simulink model "ddc_bpm_476_066"  (Simulink 7.8)
settings: Solver=ode45  StartTime=0.0  StopTime=2e-3  RelTol=1e-3
undefined symbols (not defined in the file): decim_factor_poly_35, dt_sim, frev_476, Fs_adc, n_ch, n_ovs, R_fofb, R_sec, R_sec_cfir, R_sec_pfir, xlipgetpartsetting
libraries: xbsIndex_r4 x1436, simulink x7
(part 2 of 12)

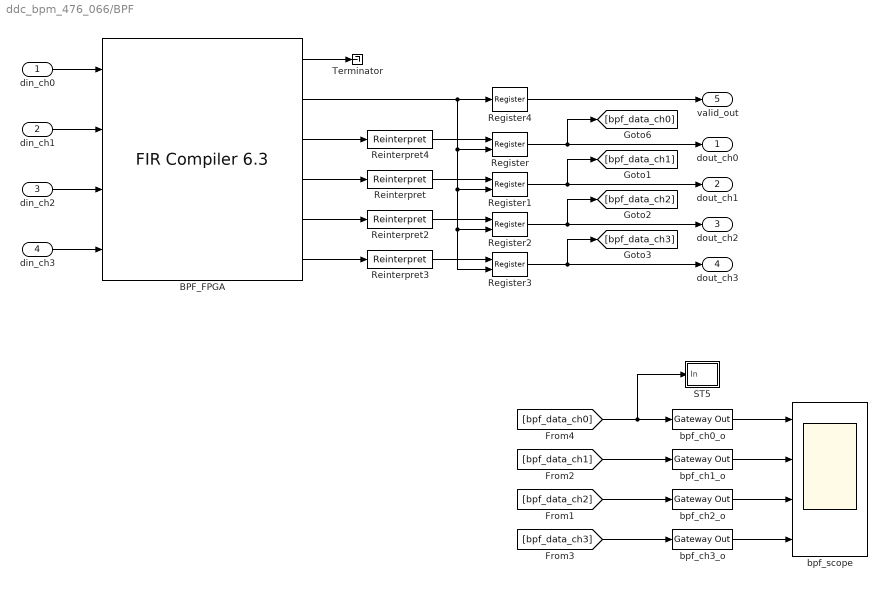
== system ddc_bpm_476_066/BPF ==
  din_ch0 : Inport
  din_ch1 : Inport  Port=2
  din_ch2 : Inport  Port=3
  din_ch3 : Inport  Port=4
  BPF_FPGA : xbsIndex_r4/FIR Compiler 6.3   coefficientvector=Hbpf_adc.Numerator  coefficient_sets=1  coefficient_reload=off  filter_type=Single_Rate  rate_change_type=Integer  interpolation_rate=1  decimation_rate=1  zero_pack_factor=1  channel_sequence=Basic  number_channels=1  pattern_list='P4-0,P4-1,P4-2,P4-3,P4-4'  number_paths=4  ratespecification=Hardware_Oversampling_Rate  sampleperiod=2  hardwareoversamplingrate=n_ovs  coefficient_sign=Signed  quantization=Quantize_Only  coefficient_width=16  bestprecision=on  coefficient_fractional_bits=17  coefficient_structure=Inferred  output_rounding_mode=Convergent_Rounding_to_Even  output_width=24  filter_architecture=Systolic_Multiply_Accumulate  optimization_goal=Area  data_buffer_type=Automatic  coefficient_buffer_type=Automatic  input_buffer_type=Automatic  output_buffer_type=Automatic  preference_for_other_storage=Automatic  multi_column_support=Automatic  columnconfig='10'  inter_column_pipe_length=4  data_has_tlast=Not_Required  m_data_has_tready=off  s_data_has_fifo=off  s_data_has_tuser=Not_Required  m_data_has_tuser=Not_Required  s_config_sync_mode=On_Vector  s_config_method=Single  num_reload_slots=1  has_aclken=off  has_aresetn=off  infoeditControl=ARESETn must be asserted for a minmum of 2 cycles  trim_axipin_name=on  passband_min=0.0  passband_max=0.5  stopband_min=0.5  stopband_max=1.0  filter_selection=1  gui_behaviour=Sysgen_GUI  data_sign=Signed  data_width=16  data_fractional_bits=0  data_tuser_width=1  wrapper_available=true  ip_wrap_arbitrary_binary_point=true  simulation_type=external_xfix  simulation_model=firv6_3_CModel:firv6_3_cmodel  ip_name=FIR Compiler  ip_version=6.3  dsptool_ready=true  ipcore_usecache=true  ipcore_useipmodelcache=true  ipcore_xco_need_fpga_part=true  port_translation_map={ 'aclken' => 'en', 'aresetn' => 'rst' }  run_core_at_system_period=true  ipcore_fpga_part=xlipgetpartsetting(gcb, {'virtex6', 'xc6vlx75t', '-3', 'ff784'})  block_type=fir_compiler_v6_3
      settings: infoedit=Maximum Possible : Maximizes oversampling rate. Abstracted input handshake (no s_data_tvalid) and automatic rate propagation.<br>Hardware Oversampling Rate : Specifies oversampling rate relative to the input sample period. Abstracted input handshake (no s_data_tvalid) and automatic rate propagation.<br>Sample Period : Specifies absolute oversampling rate. No input handshake abstraction (exposes s_data_tvalid) and no rate propagation.
  Register{,1..3} (4 alike) : xbsIndex_r4/Register  init=0  rst=off  en=on  dbl_ovrd=off  block_type=register
  Register4 : xbsIndex_r4/Register  init=0  rst=off  en=off  dbl_ovrd=off  block_type=register
  Reinterpret{,2..4} (4 alike) : xbsIndex_r4/Reinterpret  force_arith_type=off  arith_type=Unsigned  force_bin_pt=on  bin_pt=22  block_type=reinterpret
  ST5 : Subsystem
  Terminator : Terminator
  bpf_ch0_o : xbsIndex_r4/Gateway Out  inherit_from_input=on  hdl_port=on  timing_constraint=Data Rate  locs_specified=off  LOCs={}  UseAsDAC=off  DACChannel='1'  block_type=gatewayout
      settings: infoedit="Gateway out block.  Converts Xilinx fixed-point or floating-point type inputs into ouputs of type Simulink integer, single, double, or fixed point.<br><br>Hardware notes:  In hardware these blocks become top level output ports or are discarded, depending on how they are configured."
  bpf_ch1_o : xbsIndex_r4/Gateway Out  inherit_from_input=on  hdl_port=on  timing_constraint=Data Rate  locs_specified=off  LOCs={}  UseAsDAC=off  DACChannel='1'  block_type=gatewayout
      settings: infoedit="Gateway out block.  Converts Xilinx fixed-point or floating-point type inputs into ouputs of type Simulink integer, single, double, or fixed point.<br><br>Hardware notes:  In hardware these blocks become top level output ports or are discarded, depending on how they are configured."
  bpf_ch2_o : xbsIndex_r4/Gateway Out  inherit_from_input=on  hdl_port=on  timing_constraint=Data Rate  locs_specified=off  LOCs={}  UseAsDAC=off  DACChannel='1'  block_type=gatewayout
      settings: infoedit="Gateway out block.  Converts Xilinx fixed-point or floating-point type inputs into ouputs of type Simulink integer, single, double, or fixed point.<br><br>Hardware notes:  In hardware these blocks become top level output ports or are discarded, depending on how they are configured."
  bpf_ch3_o : xbsIndex_r4/Gateway Out  inherit_from_input=on  hdl_port=on  timing_constraint=Data Rate  locs_specified=off  LOCs={}  UseAsDAC=off  DACChannel='1'  block_type=gatewayout
      settings: infoedit="Gateway out block.  Converts Xilinx fixed-point or floating-point type inputs into ouputs of type Simulink integer, single, double, or fixed point.<br><br>Hardware notes:  In hardware these blocks become top level output ports or are discarded, depending on how they are configured."
  bpf_scope : Scope  NumInputPorts=4
      settings: TimeRange=0.00011214  YMin=-0.1~-1.5~-0.002~-1.5  YMax=1~1.5~0.00075~1.5  SaveName=ScopeData16  MaxDataPoints=1000000  SampleInput=on
  dout_ch0 : Outport
  dout_ch1 : Outport  Port=2
  dout_ch2 : Outport  Port=3
  dout_ch3 : Outport  Port=4
  valid_out : Outport  Port=5
  wires:
  din_ch0/1 -> BPF_FPGA/1
  BPF_FPGA/1 -> Terminator/1
  BPF_FPGA/2 -> Register/2, Register1/2, Register2/2, Register3/2, Register4/1
  BPF_FPGA/3 -> Reinterpret4/1
  BPF_FPGA/5 -> Reinterpret2/1
  din_ch1/1 -> BPF_FPGA/2
  BPF_FPGA/4 -> Reinterpret/1
  bpf_ch3_o/1 -> bpf_scope/4
  bpf_ch2_o/1 -> bpf_scope/3
  bpf_ch1_o/1 -> bpf_scope/2
  bpf_ch0_o/1 -> bpf_scope/1
  din_ch2/1 -> BPF_FPGA/3
  din_ch3/1 -> BPF_FPGA/4
  BPF_FPGA/6 -> Reinterpret3/1
  [bpf_data_ch0] -> bpf_ch0_o/1, ST5/1(In)
  [bpf_data_ch1] -> bpf_ch1_o/1
  [bpf_data_ch3] -> bpf_ch3_o/1
  [bpf_data_ch2] -> bpf_ch2_o/1
  Register/1 -> dout_ch0/1, [bpf_data_ch0]
  Register1/1 -> dout_ch1/1, [bpf_data_ch1]
  Reinterpret4/1 -> Register/1
  Reinterpret/1 -> Register1/1
  Reinterpret2/1 -> Register2/1
  Reinterpret3/1 -> Register3/1
  Register2/1 -> dout_ch2/1, [bpf_data_ch2]
  Register3/1 -> dout_ch3/1, [bpf_data_ch3]
  Register4/1 -> valid_out/1

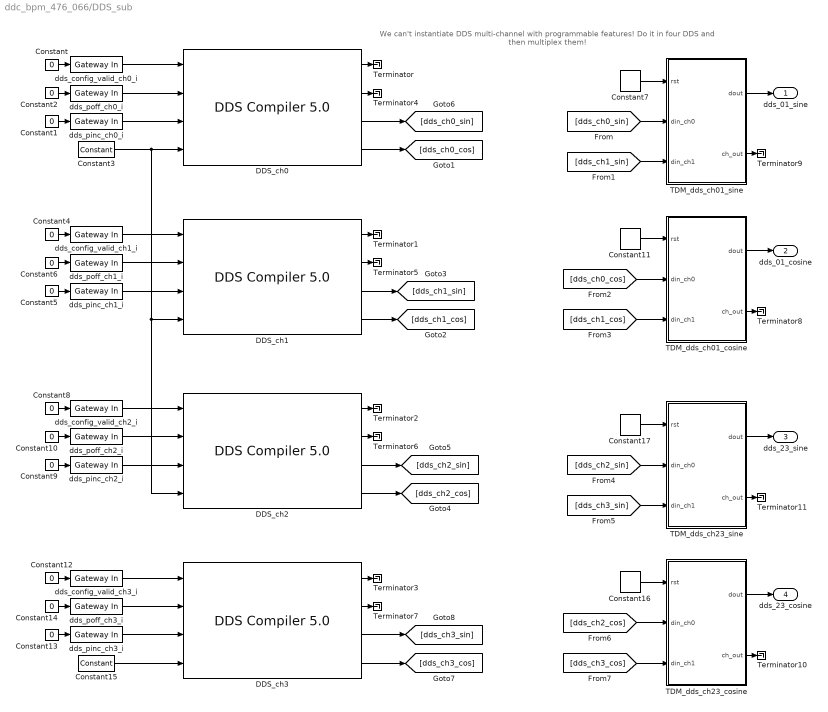
== system ddc_bpm_476_066/DDS_sub ==
  note: We can't instantiate DDS multi-channel with programmable features!
      | Do it in four DDS and then multiplex them!
  Constant{,1..2,4..6,8..10,12..14} (12 alike) : Constant  Value=0
  Constant{7,11,16..17} (4 alike) : xbsIndex_r4/Constant  const=0  gui_display_data_type=Boolean  arith_type=Boolean  n_bits=16  bin_pt=14  preci_type=Single  exp_width=8  frac_width=24  explicit_period=on  period=1/Fs_adc/n_ovs  equ=P=C  opselect=C  inp2=PCIN>>17  opr=+  inp1=P  carry=CIN  dbl_ovrd=off  block_type=constant
  Constant15 : xbsIndex_r4/Constant  const=1  gui_display_data_type=Boolean  arith_type=Boolean  n_bits=24  bin_pt=22  preci_type=Single  exp_width=8  frac_width=24  explicit_period=on  period=1/Fs_adc  equ=P=C  opselect=C  inp2=PCIN>>17  opr=+  inp1=P  carry=CIN  dbl_ovrd=off  block_type=constant
  Constant3 : xbsIndex_r4/Constant  const=1  gui_display_data_type=Boolean  arith_type=Boolean  n_bits=24  bin_pt=22  preci_type=Single  exp_width=8  frac_width=24  explicit_period=on  period=1/Fs_adc  equ=P=C  opselect=C  inp2=PCIN>>17  opr=+  inp1=P  carry=CIN  dbl_ovrd=off  block_type=constant
  DDS_ch{0..3} (4 alike) : xbsIndex_r4/DDS Compiler 5.0   partspresent=Phase_Generator_and_SIN_COS_LUT  dds_clock_rate=Fs_adc/1e6  channels=1  parameter_entry=Hardware_Parameters  spurious_free_dynamic_range=36  frequency_resolution=0.4  noise_shaping=Taylor_Series_Corrected  phase_width=30  output_width=24  output_selection=Sine_and_Cosine  negative_sine=on  negative_cosine=off  amplitude_mode=Unit_Circle  memory_type=Auto  optimization_goal=Auto  dsp48_use=Minimal  latency_configuration=Auto  latency=12  has_phase_out=off  has_aclken=off  has_aresetn=off  explicit_period=on  period=1/Fs_adc  data_has_tlast=Not_Required  has_tready=on  s_phase_has_tuser=Not_Required  m_data_has_tuser=Not_Required  m_phase_has_tuser=Not_Required  s_phase_tuser_width=1  s_config_sync_mode=On_Vector  phase_increment=Programmable  output_frequency1=0  output_frequency2=0  output_frequency3=0  output_frequency4=0  output_frequency5=0  output_frequency6=0  output_frequency7=0  output_frequency8=0  output_frequency9=0  output_frequency10=0  output_frequency11=0  output_frequency12=0  output_frequency13=0  output_frequency14=0  output_frequency15=0  output_frequency16=0  pinc1=dds_freq_bin  pinc2='0'  pinc3='0'  pinc4='0'  pinc5='0'  pinc6='0'  pinc7='0'  pinc8='0'  pinc9='0'  pinc10='0'  pinc11='0'  pinc12='0'  pinc13='0'  pinc14='0'  pinc15='0'  pinc16='0'  phase_offset=Programmable  phase_offset_angles1=0  phase_offset_angles2=0  phase_offset_angles3=0  phase_offset_angles4=0  phase_offset_angles5=0  phase_offset_angles6=0  phase_offset_angles7=0  phase_offset_angles8=0  phase_offset_angles9=0  phase_offset_angles10=0  phase_offset_angles11=0  phase_offset_angles12=0  phase_offset_angles13=0  phase_offset_angles14=0  phase_offset_angles15=0  phase_offset_angles16=0  poff1='0'  poff2='0'  poff3='0'  poff4='0'  poff5='0'  poff6='0'  poff7='0'  poff8='0'  poff9='0'  poff10='0'  poff11='0'  poff12='0'  poff13='0'  poff14='0'  poff15='0'  poff16='0'  trim_axipin_name=on  por_mode=false  gui_behaviour=Sysgen  ip_name=DDS Compiler  ip_version=5.0  dsptool_ready=true  wrapper_available=true  port_translation_map={ 'aclken' => 'en', 'aresetn' => 'rst' }  ipcore_xco_need_fpga_part=true  ipcore_fpga_part=xlipgetpartsetting(gcb, {'virtex6', 'xc6vlx75t', '-3', 'ff784'})  ipcore_usecache=true  ipcore_useipmodelcache=true  ipcore_verbose=false  block_type=dds_compiler_v5_0
  TDM_dds_ch01_cosine : Subsystem
  TDM_dds_ch01_sine : Subsystem
  TDM_dds_ch23_cosine : Subsystem
  TDM_dds_ch23_sine : Subsystem
  Terminator{,1..11} (12 alike) : Terminator
  dds_config_valid_ch0_i : xbsIndex_r4/Gateway In  gui_display_data_type=Boolean  arith_type=Boolean  n_bits=16  bin_pt=15  preci_type=Single  exp_width=8  frac_width=24  quantization=Truncate  overflow=Flag as error  period=1/Fs_adc  dbl_ovrd=off  timing_constraint=None  locs_specified=off  LOCs={}  inherit_from_input=off  UseAsADC=off  ADCChannel='1'  hdl_port=on  block_type=gatewayin
      settings: infoedit="Gateway in block.  Converts inputs of type Simulink integer, single, double and fixed point to  Xilinx fixed-point or floating-point data type.<br><br>Hardware notes:  In hardware these blocks become top level input ports."
  dds_config_valid_ch1_i : xbsIndex_r4/Gateway In  gui_display_data_type=Boolean  arith_type=Boolean  n_bits=16  bin_pt=15  preci_type=Single  exp_width=8  frac_width=24  quantization=Truncate  overflow=Flag as error  period=1/Fs_adc  dbl_ovrd=off  timing_constraint=None  locs_specified=off  LOCs={}  inherit_from_input=off  UseAsADC=off  ADCChannel='1'  hdl_port=on  block_type=gatewayin
      settings: infoedit="Gateway in block.  Converts inputs of type Simulink integer, single, double and fixed point to  Xilinx fixed-point or floating-point data type.<br><br>Hardware notes:  In hardware these blocks become top level input ports."
  dds_config_valid_ch2_i : xbsIndex_r4/Gateway In  gui_display_data_type=Boolean  arith_type=Boolean  n_bits=16  bin_pt=15  preci_type=Single  exp_width=8  frac_width=24  quantization=Truncate  overflow=Flag as error  period=1/Fs_adc  dbl_ovrd=off  timing_constraint=None  locs_specified=off  LOCs={}  inherit_from_input=off  UseAsADC=off  ADCChannel='1'  hdl_port=on  block_type=gatewayin
      settings: infoedit="Gateway in block.  Converts inputs of type Simulink integer, single, double and fixed point to  Xilinx fixed-point or floating-point data type.<br><br>Hardware notes:  In hardware these blocks become top level input ports."
  dds_config_valid_ch3_i : xbsIndex_r4/Gateway In  gui_display_data_type=Boolean  arith_type=Boolean  n_bits=16  bin_pt=15  preci_type=Single  exp_width=8  frac_width=24  quantization=Truncate  overflow=Flag as error  period=1/Fs_adc  dbl_ovrd=off  timing_constraint=None  locs_specified=off  LOCs={}  inherit_from_input=off  UseAsADC=off  ADCChannel='1'  hdl_port=on  block_type=gatewayin
      settings: infoedit="Gateway in block.  Converts inputs of type Simulink integer, single, double and fixed point to  Xilinx fixed-point or floating-point data type.<br><br>Hardware notes:  In hardware these blocks become top level input ports."
  dds_pinc_ch0_i : xbsIndex_r4/Gateway In  gui_display_data_type=Fixed-point  arith_type="Signed  (2's comp)"  n_bits=30  bin_pt=30  preci_type=Single  exp_width=8  frac_width=24  quantization=Truncate  overflow=Flag as error  period=1/Fs_adc  dbl_ovrd=off  timing_constraint=None  locs_specified=off  LOCs={}  inherit_from_input=off  UseAsADC=off  ADCChannel='1'  hdl_port=on  block_type=gatewayin
      settings: infoedit="Gateway in block.  Converts inputs of type Simulink integer, single, double and fixed point to  Xilinx fixed-point or floating-point data type.<br><br>Hardware notes:  In hardware these blocks become top level input ports."
  dds_pinc_ch1_i : xbsIndex_r4/Gateway In  gui_display_data_type=Fixed-point  arith_type="Signed  (2's comp)"  n_bits=30  bin_pt=30  preci_type=Single  exp_width=8  frac_width=24  quantization=Truncate  overflow=Flag as error  period=1/Fs_adc  dbl_ovrd=off  timing_constraint=None  locs_specified=off  LOCs={}  inherit_from_input=off  UseAsADC=off  ADCChannel='1'  hdl_port=on  block_type=gatewayin
      settings: infoedit="Gateway in block.  Converts inputs of type Simulink integer, single, double and fixed point to  Xilinx fixed-point or floating-point data type.<br><br>Hardware notes:  In hardware these blocks become top level input ports."
  dds_pinc_ch2_i : xbsIndex_r4/Gateway In  gui_display_data_type=Fixed-point  arith_type="Signed  (2's comp)"  n_bits=30  bin_pt=30  preci_type=Single  exp_width=8  frac_width=24  quantization=Truncate  overflow=Flag as error  period=1/Fs_adc  dbl_ovrd=off  timing_constraint=None  locs_specified=off  LOCs={}  inherit_from_input=off  UseAsADC=off  ADCChannel='1'  hdl_port=on  block_type=gatewayin
      settings: infoedit="Gateway in block.  Converts inputs of type Simulink integer, single, double and fixed point to  Xilinx fixed-point or floating-point data type.<br><br>Hardware notes:  In hardware these blocks become top level input ports."
  dds_pinc_ch3_i : xbsIndex_r4/Gateway In  gui_display_data_type=Fixed-point  arith_type="Signed  (2's comp)"  n_bits=30  bin_pt=30  preci_type=Single  exp_width=8  frac_width=24  quantization=Truncate  overflow=Flag as error  period=1/Fs_adc  dbl_ovrd=off  timing_constraint=None  locs_specified=off  LOCs={}  inherit_from_input=off  UseAsADC=off  ADCChannel='1'  hdl_port=on  block_type=gatewayin
      settings: infoedit="Gateway in block.  Converts inputs of type Simulink integer, single, double and fixed point to  Xilinx fixed-point or floating-point data type.<br><br>Hardware notes:  In hardware these blocks become top level input ports."
  dds_poff_ch0_i : xbsIndex_r4/Gateway In  gui_display_data_type=Fixed-point  arith_type="Signed  (2's comp)"  n_bits=30  bin_pt=30  preci_type=Single  exp_width=8  frac_width=24  quantization=Truncate  overflow=Flag as error  period=1/Fs_adc  dbl_ovrd=off  timing_constraint=None  locs_specified=off  LOCs={}  inherit_from_input=off  UseAsADC=off  ADCChannel='1'  hdl_port=on  block_type=gatewayin
      settings: infoedit="Gateway in block.  Converts inputs of type Simulink integer, single, double and fixed point to  Xilinx fixed-point or floating-point data type.<br><br>Hardware notes:  In hardware these blocks become top level input ports."
  dds_poff_ch1_i : xbsIndex_r4/Gateway In  gui_display_data_type=Fixed-point  arith_type="Signed  (2's comp)"  n_bits=30  bin_pt=30  preci_type=Single  exp_width=8  frac_width=24  quantization=Truncate  overflow=Flag as error  period=1/Fs_adc  dbl_ovrd=off  timing_constraint=None  locs_specified=off  LOCs={}  inherit_from_input=off  UseAsADC=off  ADCChannel='1'  hdl_port=on  block_type=gatewayin
      settings: infoedit="Gateway in block.  Converts inputs of type Simulink integer, single, double and fixed point to  Xilinx fixed-point or floating-point data type.<br><br>Hardware notes:  In hardware these blocks become top level input ports."
  dds_poff_ch2_i : xbsIndex_r4/Gateway In  gui_display_data_type=Fixed-point  arith_type="Signed  (2's comp)"  n_bits=30  bin_pt=30  preci_type=Single  exp_width=8  frac_width=24  quantization=Truncate  overflow=Flag as error  period=1/Fs_adc  dbl_ovrd=off  timing_constraint=None  locs_specified=off  LOCs={}  inherit_from_input=off  UseAsADC=off  ADCChannel='1'  hdl_port=on  block_type=gatewayin
      settings: infoedit="Gateway in block.  Converts inputs of type Simulink integer, single, double and fixed point to  Xilinx fixed-point or floating-point data type.<br><br>Hardware notes:  In hardware these blocks become top level input ports."
  dds_poff_ch3_i : xbsIndex_r4/Gateway In  gui_display_data_type=Fixed-point  arith_type="Signed  (2's comp)"  n_bits=30  bin_pt=30  preci_type=Single  exp_width=8  frac_width=24  quantization=Truncate  overflow=Flag as error  period=1/Fs_adc  dbl_ovrd=off  timing_constraint=None  locs_specified=off  LOCs={}  inherit_from_input=off  UseAsADC=off  ADCChannel='1'  hdl_port=on  block_type=gatewayin
      settings: infoedit="Gateway in block.  Converts inputs of type Simulink integer, single, double and fixed point to  Xilinx fixed-point or floating-point data type.<br><br>Hardware notes:  In hardware these blocks become top level input ports."
  dds_01_sine : Outport
  dds_01_cosine : Outport  Port=2
  dds_23_sine : Outport  Port=3
  dds_23_cosine : Outport  Port=4
  wires:
  Constant3/1 -> DDS_ch0/4, DDS_ch1/4, DDS_ch2/4
  dds_poff_ch0_i/1 -> DDS_ch0/2
  dds_pinc_ch0_i/1 -> DDS_ch0/3
  dds_config_valid_ch0_i/1 -> DDS_ch0/1
  DDS_ch0/1 -> Terminator/1
  Constant/1 -> dds_config_valid_ch0_i/1
  Constant1/1 -> dds_pinc_ch0_i/1
  Constant2/1 -> dds_poff_ch0_i/1
  dds_poff_ch1_i/1 -> DDS_ch1/2
  dds_pinc_ch1_i/1 -> DDS_ch1/3
  dds_config_valid_ch1_i/1 -> DDS_ch1/1
  DDS_ch1/1 -> Terminator1/1
  Constant4/1 -> dds_config_valid_ch1_i/1
  Constant5/1 -> dds_pinc_ch1_i/1
  Constant6/1 -> dds_poff_ch1_i/1
  dds_poff_ch2_i/1 -> DDS_ch2/2
  dds_pinc_ch2_i/1 -> DDS_ch2/3
  dds_config_valid_ch2_i/1 -> DDS_ch2/1
  DDS_ch2/1 -> Terminator2/1
  Constant8/1 -> dds_config_valid_ch2_i/1
  Constant9/1 -> dds_pinc_ch2_i/1
  Constant10/1 -> dds_poff_ch2_i/1
  Constant15/1 -> DDS_ch3/4
  dds_poff_ch3_i/1 -> DDS_ch3/2
  dds_pinc_ch3_i/1 -> DDS_ch3/3
  dds_config_valid_ch3_i/1 -> DDS_ch3/1
  DDS_ch3/1 -> Terminator3/1
  Constant12/1 -> dds_config_valid_ch3_i/1
  Constant13/1 -> dds_pinc_ch3_i/1
  Constant14/1 -> dds_poff_ch3_i/1
  Constant7/1 -> TDM_dds_ch01_sine/1(rst)
  TDM_dds_ch01_sine/1(dout) -> dds_01_sine/1
  Constant11/1 -> TDM_dds_ch01_cosine/1(rst)
  TDM_dds_ch01_cosine/1(dout) -> dds_01_cosine/1
  DDS_ch0/3 -> [dds_ch0_sin]
  DDS_ch0/4 -> [dds_ch0_cos]
  DDS_ch1/3 -> [dds_ch1_sin]
  DDS_ch1/4 -> [dds_ch1_cos]
  DDS_ch2/3 -> [dds_ch2_sin]
  DDS_ch2/4 -> [dds_ch2_cos]
  DDS_ch3/3 -> [dds_ch3_sin]
  DDS_ch3/4 -> [dds_ch3_cos]
  [dds_ch0_sin] -> TDM_dds_ch01_sine/2(din_ch0)
  [dds_ch1_sin] -> TDM_dds_ch01_sine/3(din_ch1)
  [dds_ch0_cos] -> TDM_dds_ch01_cosine/2(din_ch0)
  [dds_ch1_cos] -> TDM_dds_ch01_cosine/3(din_ch1)
  Constant17/1 -> TDM_dds_ch23_sine/1(rst)
  TDM_dds_ch23_sine/1(dout) -> dds_23_sine/1
  Constant16/1 -> TDM_dds_ch23_cosine/1(rst)
  TDM_dds_ch23_cosine/1(dout) -> dds_23_cosine/1
  [dds_ch2_sin] -> TDM_dds_ch23_sine/2(din_ch0)
  [dds_ch3_sin] -> TDM_dds_ch23_sine/3(din_ch1)
  [dds_ch2_cos] -> TDM_dds_ch23_cosine/2(din_ch0)
  [dds_ch3_cos] -> TDM_dds_ch23_cosine/3(din_ch1)
  DDS_ch0/2 -> Terminator4/1
  DDS_ch1/2 -> Terminator5/1
  DDS_ch2/2 -> Terminator6/1
  DDS_ch3/2 -> Terminator7/1
  TDM_dds_ch01_cosine/2(ch_out) -> Terminator8/1
  TDM_dds_ch01_sine/2(ch_out) -> Terminator9/1
  TDM_dds_ch23_cosine/2(ch_out) -> Terminator10/1
  TDM_dds_ch23_sine/2(ch_out) -> Terminator11/1

== system ddc_bpm_476_066/FOFB_amp ==
  Q_in0 : Inport
  I_in0 : Inport  Port=2
  ch_in0 : Inport  Port=3
  Q_in1 : Inport  Port=4
  I_in1 : Inport  Port=5
  ch_in1 : Inport  Port=6
  ST1 : Subsystem
  ST5 : Subsystem
  TDDM_fofb_amp_4ch : Subsystem
  Terminator{,1..3} (4 alike) : Terminator
  fofb_amp0 : Subsystem
  fofb_amp1 : Subsystem
  amp_out0 : Outport
  amp_out1 : Outport  Port=2
  amp_out2 : Outport  Port=3
  amp_out3 : Outport  Port=4
  wires:
  Q_in0/1 -> fofb_amp0/1(Q_in)
  I_in0/1 -> fofb_amp0/2(I_in)
  ch_in0/1 -> fofb_amp0/3(ch_in)
  Q_in1/1 -> fofb_amp1/1(Q_in)
  I_in1/1 -> fofb_amp1/2(I_in)
  ch_in1/1 -> fofb_amp1/3(ch_in)
  TDDM_fofb_amp_4ch/1(amp_out0) -> amp_out0/1, ST1/1(In)
  TDDM_fofb_amp_4ch/2(amp_out1) -> amp_out1/1
  TDDM_fofb_amp_4ch/3(amp_out2) -> amp_out2/1
  TDDM_fofb_amp_4ch/4(amp_out3) -> amp_out3/1
  fofb_amp0/1(amp_out) -> TDDM_fofb_amp_4ch/1(amp_in0), ST5/1(In)
  fofb_amp0/4(ch_out) -> TDDM_fofb_amp_4ch/2(ch_in0)
  fofb_amp1/1(amp_out) -> TDDM_fofb_amp_4ch/3(amp_in1)
  fofb_amp1/4(ch_out) -> TDDM_fofb_amp_4ch/4(ch_in1)
  fofb_amp0/2(phase_out) -> Terminator/1
  fofb_amp0/3(valid_out) -> Terminator1/1
  fofb_amp1/2(phase_out) -> Terminator2/1
  fofb_amp1/3(valid_out) -> Terminator3/1

== system ddc_bpm_476_066/K_fofb_mult3 ==
  In1 : Inport
  In2 : Inport  Port=2
  vld_in : Inport  Port=3
  Cast_truncate1 : Subsystem
  Delay1 : xbsIndex_r4/Delay  rst=off  infoeditControl=Selection of Reset will increase slice count due to use of real FFs and instead of SRLs  en=off  latency=9  dbl_ovrd=off  reg_retiming=off  block_type=delay
  Kx_tbt : xbsIndex_r4/Mult  precision=Full  arith_type="Signed  (2's comp)"  n_bits=16  bin_pt=14  quantization=Truncate  overflow=Wrap  en=off  latency=8  dbl_ovrd=off  use_behavioral_HDL=off  opt=Speed  use_embedded=off  optimum_pipeline=on  pipeline=on  use_rpm=on  placement_style=Triangular  block_type=mult
  Register : xbsIndex_r4/Register  init=0  rst=off  en=off  dbl_ovrd=off  block_type=register
  Out1 : Outport
  vld_out : Outport  Port=2
  wires:
  Kx_tbt/1 -> Cast_truncate1/1(In1)
  In1/1 -> Kx_tbt/1
  Cast_truncate1/1(Out1) -> Register/1
  In2/1 -> Kx_tbt/2
  Register/1 -> Out1/1
  vld_in/1 -> Delay1/1
  Delay1/1 -> vld_out/1

== system ddc_bpm_476_066/K_fofb_mult4 ==
  In1 : Inport
  In2 : Inport  Port=2
  vld_in : Inport  Port=3
  Cast_truncate1 : Subsystem
  Delay1 : xbsIndex_r4/Delay  rst=off  infoeditControl=Selection of Reset will increase slice count due to use of real FFs and instead of SRLs  en=off  latency=9  dbl_ovrd=off  reg_retiming=off  block_type=delay
  Kx_tbt : xbsIndex_r4/Mult  precision=Full  arith_type="Signed  (2's comp)"  n_bits=16  bin_pt=14  quantization=Truncate  overflow=Wrap  en=off  latency=8  dbl_ovrd=off  use_behavioral_HDL=off  opt=Speed  use_embedded=off  optimum_pipeline=on  pipeline=on  use_rpm=on  placement_style=Triangular  block_type=mult
  Register : xbsIndex_r4/Register  init=0  rst=off  en=off  dbl_ovrd=off  block_type=register
  Out1 : Outport
  vld_out : Outport  Port=2
  wires:
  Kx_tbt/1 -> Cast_truncate1/1(In1)
  In1/1 -> Kx_tbt/1
  Cast_truncate1/1(Out1) -> Register/1
  In2/1 -> Kx_tbt/2
  Register/1 -> Out1/1
  vld_in/1 -> Delay1/1
  Delay1/1 -> vld_out/1

== system ddc_bpm_476_066/K_fofb_mult5 ==
  In1 : Inport
  In2 : Inport  Port=2
  vld_in : Inport  Port=3
  Cast_truncate1 : Subsystem
  Delay1 : xbsIndex_r4/Delay  rst=off  infoeditControl=Selection of Reset will increase slice count due to use of real FFs and instead of SRLs  en=off  latency=9  dbl_ovrd=off  reg_retiming=off  block_type=delay
  Kx_tbt : xbsIndex_r4/Mult  precision=Full  arith_type="Signed  (2's comp)"  n_bits=16  bin_pt=14  quantization=Truncate  overflow=Wrap  en=off  latency=8  dbl_ovrd=off  use_behavioral_HDL=off  opt=Speed  use_embedded=off  optimum_pipeline=on  pipeline=on  use_rpm=on  placement_style=Triangular  block_type=mult
  Register : xbsIndex_r4/Register  init=0  rst=off  en=off  dbl_ovrd=off  block_type=register
  Out1 : Outport
  vld_out : Outport  Port=2
  wires:
  Kx_tbt/1 -> Cast_truncate1/1(In1)
  In1/1 -> Kx_tbt/1
  Cast_truncate1/1(Out1) -> Register/1
  In2/1 -> Kx_tbt/2
  Register/1 -> Out1/1
  vld_in/1 -> Delay1/1
  Delay1/1 -> vld_out/1

== system ddc_bpm_476_066/K_monit_1_mult ==
  In1 : Inport
  In2 : Inport  Port=2
  vld_in : Inport  Port=3
  Cast_truncate1 : Subsystem
  Delay1 : xbsIndex_r4/Delay  rst=off  infoeditControl=Selection of Reset will increase slice count due to use of real FFs and instead of SRLs  en=off  latency=9  dbl_ovrd=off  reg_retiming=off  block_type=delay
  Kx_tbt : xbsIndex_r4/Mult  precision=Full  arith_type="Signed  (2's comp)"  n_bits=16  bin_pt=14  quantization=Truncate  overflow=Wrap  en=off  latency=8  dbl_ovrd=off  use_behavioral_HDL=off  opt=Speed  use_embedded=off  optimum_pipeline=on  pipeline=on  use_rpm=on  placement_style=Triangular  block_type=mult
  Register : xbsIndex_r4/Register  init=0  rst=off  en=off  dbl_ovrd=off  block_type=register
  Out1 : Outport
  vld_out : Outport  Port=2
  wires:
  Kx_tbt/1 -> Cast_truncate1/1(In1)
  In1/1 -> Kx_tbt/1
  Cast_truncate1/1(Out1) -> Register/1
  In2/1 -> Kx_tbt/2
  Register/1 -> Out1/1
  vld_in/1 -> Delay1/1
  Delay1/1 -> vld_out/1

== system ddc_bpm_476_066/K_monit_1_mult2 ==
  In1 : Inport
  In2 : Inport  Port=2
  vld_in : Inport  Port=3
  Cast_truncate1 : Subsystem
  Delay1 : xbsIndex_r4/Delay  rst=off  infoeditControl=Selection of Reset will increase slice count due to use of real FFs and instead of SRLs  en=off  latency=9  dbl_ovrd=off  reg_retiming=off  block_type=delay
  Kx_tbt : xbsIndex_r4/Mult  precision=Full  arith_type="Signed  (2's comp)"  n_bits=16  bin_pt=14  quantization=Truncate  overflow=Wrap  en=off  latency=8  dbl_ovrd=off  use_behavioral_HDL=off  opt=Speed  use_embedded=off  optimum_pipeline=on  pipeline=on  use_rpm=on  placement_style=Triangular  block_type=mult
  Register : xbsIndex_r4/Register  init=0  rst=off  en=off  dbl_ovrd=off  block_type=register
  Out1 : Outport
  vld_out : Outport  Port=2
  wires:
  Kx_tbt/1 -> Cast_truncate1/1(In1)
  In1/1 -> Kx_tbt/1
  Cast_truncate1/1(Out1) -> Register/1
  In2/1 -> Kx_tbt/2
  Register/1 -> Out1/1
  vld_in/1 -> Delay1/1
  Delay1/1 -> vld_out/1

== system ddc_bpm_476_066/K_monit_1_mult6 ==
  In1 : Inport
  In2 : Inport  Port=2
  vld_in : Inport  Port=3
  Cast_truncate1 : Subsystem
  Delay1 : xbsIndex_r4/Delay  rst=off  infoeditControl=Selection of Reset will increase slice count due to use of real FFs and instead of SRLs  en=off  latency=9  dbl_ovrd=off  reg_retiming=off  block_type=delay
  Kx_tbt : xbsIndex_r4/Mult  precision=Full  arith_type="Signed  (2's comp)"  n_bits=16  bin_pt=14  quantization=Truncate  overflow=Wrap  en=off  latency=8  dbl_ovrd=off  use_behavioral_HDL=off  opt=Speed  use_embedded=off  optimum_pipeline=on  pipeline=on  use_rpm=on  placement_style=Triangular  block_type=mult
  Register : xbsIndex_r4/Register  init=0  rst=off  en=off  dbl_ovrd=off  block_type=register
  Out1 : Outport
  vld_out : Outport  Port=2
  wires:
  Kx_tbt/1 -> Cast_truncate1/1(In1)
  In1/1 -> Kx_tbt/1
  Cast_truncate1/1(Out1) -> Register/1
  In2/1 -> Kx_tbt/2
  Register/1 -> Out1/1
  vld_in/1 -> Delay1/1
  Delay1/1 -> vld_out/1

== system ddc_bpm_476_066/K_monit_mult3 ==
  In1 : Inport
  In2 : Inport  Port=2
  vld_in : Inport  Port=3
  Cast_truncate1 : Subsystem
  Delay1 : xbsIndex_r4/Delay  rst=off  infoeditControl=Selection of Reset will increase slice count due to use of real FFs and instead of SRLs  en=off  latency=9  dbl_ovrd=off  reg_retiming=off  block_type=delay
  Kx_tbt : xbsIndex_r4/Mult  precision=Full  arith_type="Signed  (2's comp)"  n_bits=16  bin_pt=14  quantization=Truncate  overflow=Wrap  en=off  latency=8  dbl_ovrd=off  use_behavioral_HDL=off  opt=Speed  use_embedded=off  optimum_pipeline=on  pipeline=on  use_rpm=on  placement_style=Triangular  block_type=mult
  Register : xbsIndex_r4/Register  init=0  rst=off  en=off  dbl_ovrd=off  block_type=register
  Out1 : Outport
  vld_out : Outport  Port=2
  wires:
  Kx_tbt/1 -> Cast_truncate1/1(In1)
  In1/1 -> Kx_tbt/1
  Cast_truncate1/1(Out1) -> Register/1
  In2/1 -> Kx_tbt/2
  Register/1 -> Out1/1
  vld_in/1 -> Delay1/1
  Delay1/1 -> vld_out/1

== system ddc_bpm_476_066/K_monit_mult4 ==
  In1 : Inport
  In2 : Inport  Port=2
  vld_in : Inport  Port=3
  Cast_truncate1 : Subsystem
  Delay1 : xbsIndex_r4/Delay  rst=off  infoeditControl=Selection of Reset will increase slice count due to use of real FFs and instead of SRLs  en=off  latency=9  dbl_ovrd=off  reg_retiming=off  block_type=delay
  Kx_tbt : xbsIndex_r4/Mult  precision=Full  arith_type="Signed  (2's comp)"  n_bits=16  bin_pt=14  quantization=Truncate  overflow=Wrap  en=off  latency=8  dbl_ovrd=off  use_behavioral_HDL=off  opt=Speed  use_embedded=off  optimum_pipeline=on  pipeline=on  use_rpm=on  placement_style=Triangular  block_type=mult
  Register : xbsIndex_r4/Register  init=0  rst=off  en=off  dbl_ovrd=off  block_type=register
  Out1 : Outport
  vld_out : Outport  Port=2
  wires:
  Kx_tbt/1 -> Cast_truncate1/1(In1)
  In1/1 -> Kx_tbt/1
  Cast_truncate1/1(Out1) -> Register/1
  In2/1 -> Kx_tbt/2
  Register/1 -> Out1/1
  vld_in/1 -> Delay1/1
  Delay1/1 -> vld_out/1

== system ddc_bpm_476_066/K_monit_mult5 ==
  In1 : Inport
  In2 : Inport  Port=2
  vld_in : Inport  Port=3
  Cast_truncate1 : Subsystem
  Delay1 : xbsIndex_r4/Delay  rst=off  infoeditControl=Selection of Reset will increase slice count due to use of real FFs and instead of SRLs  en=off  latency=9  dbl_ovrd=off  reg_retiming=off  block_type=delay
  Kx_tbt : xbsIndex_r4/Mult  precision=Full  arith_type="Signed  (2's comp)"  n_bits=16  bin_pt=14  quantization=Truncate  overflow=Wrap  en=off  latency=8  dbl_ovrd=off  use_behavioral_HDL=off  opt=Speed  use_embedded=off  optimum_pipeline=on  pipeline=on  use_rpm=on  placement_style=Triangular  block_type=mult
  Register : xbsIndex_r4/Register  init=0  rst=off  en=off  dbl_ovrd=off  block_type=register
  Out1 : Outport
  vld_out : Outport  Port=2
  wires:
  Kx_tbt/1 -> Cast_truncate1/1(In1)
  In1/1 -> Kx_tbt/1
  Cast_truncate1/1(Out1) -> Register/1
  In2/1 -> Kx_tbt/2
  Register/1 -> Out1/1
  vld_in/1 -> Delay1/1
  Delay1/1 -> vld_out/1

== system ddc_bpm_476_066/K_tbt_mult ==
  In1 : Inport
  In2 : Inport  Port=2
  vld_in : Inport  Port=3
  Cast_truncate1 : Subsystem
  Delay1 : xbsIndex_r4/Delay  rst=off  infoeditControl=Selection of Reset will increase slice count due to use of real FFs and instead of SRLs  en=off  latency=9  dbl_ovrd=off  reg_retiming=off  block_type=delay
  Kx_tbt : xbsIndex_r4/Mult  precision=Full  arith_type="Signed  (2's comp)"  n_bits=16  bin_pt=14  quantization=Truncate  overflow=Wrap  en=off  latency=8  dbl_ovrd=off  use_behavioral_HDL=off  opt=Speed  use_embedded=off  optimum_pipeline=on  pipeline=on  use_rpm=on  placement_style=Triangular  block_type=mult
  Register : xbsIndex_r4/Register  init=0  rst=off  en=off  dbl_ovrd=off  block_type=register
  Out1 : Outport
  vld_out : Outport  Port=2
  wires:
  Kx_tbt/1 -> Cast_truncate1/1(In1)
  In1/1 -> Kx_tbt/1
  Cast_truncate1/1(Out1) -> Register/1
  In2/1 -> Kx_tbt/2
  Register/1 -> Out1/1
  vld_in/1 -> Delay1/1
  Delay1/1 -> vld_out/1

== system ddc_bpm_476_066/K_tbt_mult1 ==
  In1 : Inport
  In2 : Inport  Port=2
  vld_in : Inport  Port=3
  Cast_truncate1 : Subsystem
  Delay1 : xbsIndex_r4/Delay  rst=off  infoeditControl=Selection of Reset will increase slice count due to use of real FFs and instead of SRLs  en=off  latency=9  dbl_ovrd=off  reg_retiming=off  block_type=delay
  Kx_tbt : xbsIndex_r4/Mult  precision=Full  arith_type="Signed  (2's comp)"  n_bits=16  bin_pt=14  quantization=Truncate  overflow=Wrap  en=off  latency=8  dbl_ovrd=off  use_behavioral_HDL=off  opt=Speed  use_embedded=off  optimum_pipeline=on  pipeline=on  use_rpm=on  placement_style=Triangular  block_type=mult
  Register : xbsIndex_r4/Register  init=0  rst=off  en=off  dbl_ovrd=off  block_type=register
  Out1 : Outport
  vld_out : Outport  Port=2
  wires:
  Kx_tbt/1 -> Cast_truncate1/1(In1)
  In1/1 -> Kx_tbt/1
  Cast_truncate1/1(Out1) -> Register/1
  In2/1 -> Kx_tbt/2
  Register/1 -> Out1/1
  vld_in/1 -> Delay1/1
  Delay1/1 -> vld_out/1

== system ddc_bpm_476_066/K_tbt_mult2 ==
  In1 : Inport
  In2 : Inport  Port=2
  vld_in : Inport  Port=3
  Cast_truncate1 : Subsystem
  Delay1 : xbsIndex_r4/Delay  rst=off  infoeditControl=Selection of Reset will increase slice count due to use of real FFs and instead of SRLs  en=off  latency=9  dbl_ovrd=off  reg_retiming=off  block_type=delay
  Kx_tbt : xbsIndex_r4/Mult  precision=Full  arith_type="Signed  (2's comp)"  n_bits=16  bin_pt=14  quantization=Truncate  overflow=Wrap  en=off  latency=8  dbl_ovrd=off  use_behavioral_HDL=off  opt=Speed  use_embedded=off  optimum_pipeline=on  pipeline=on  use_rpm=on  placement_style=Triangular  block_type=mult
  Register : xbsIndex_r4/Register  init=0  rst=off  en=off  dbl_ovrd=off  block_type=register
  Out1 : Outport
  vld_out : Outport  Port=2
  wires:
  Kx_tbt/1 -> Cast_truncate1/1(In1)
  In1/1 -> Kx_tbt/1
  Cast_truncate1/1(Out1) -> Register/1
  In2/1 -> Kx_tbt/2
  Register/1 -> Out1/1
  vld_in/1 -> Delay1/1
  Delay1/1 -> vld_out/1

== system ddc_bpm_476_066/Ksum_fofb_mult4 ==
  In1 : Inport
  In2 : Inport  Port=2
  vld_in : Inport  Port=3
  Cast_truncate1 : Subsystem
  Delay1 : xbsIndex_r4/Delay  rst=off  infoeditControl=Selection of Reset will increase slice count due to use of real FFs and instead of SRLs  en=off  latency=9  dbl_ovrd=off  reg_retiming=off  block_type=delay
  Kx_tbt : xbsIndex_r4/Mult  precision=Full  arith_type="Signed  (2's comp)"  n_bits=16  bin_pt=14  quantization=Truncate  overflow=Wrap  en=off  latency=8  dbl_ovrd=off  use_behavioral_HDL=off  opt=Speed  use_embedded=off  optimum_pipeline=on  pipeline=on  use_rpm=on  placement_style=Triangular  block_type=mult
  Register : xbsIndex_r4/Register  init=0  rst=off  en=off  dbl_ovrd=off  block_type=register
  Out1 : Outport
  vld_out : Outport  Port=2
  wires:
  Kx_tbt/1 -> Cast_truncate1/1(In1)
  In1/1 -> Kx_tbt/1
  Cast_truncate1/1(Out1) -> Register/1
  In2/1 -> Kx_tbt/2
  Register/1 -> Out1/1
  vld_in/1 -> Delay1/1
  Delay1/1 -> vld_out/1

== system ddc_bpm_476_066/Ksum_monit_1_mult1 ==
  In1 : Inport
  In2 : Inport  Port=2
  vld_in : Inport  Port=3
  Cast_truncate1 : Subsystem
  Delay1 : xbsIndex_r4/Delay  rst=off  infoeditControl=Selection of Reset will increase slice count due to use of real FFs and instead of SRLs  en=off  latency=9  dbl_ovrd=off  reg_retiming=off  block_type=delay
  Kx_tbt : xbsIndex_r4/Mult  precision=Full  arith_type="Signed  (2's comp)"  n_bits=16  bin_pt=14  quantization=Truncate  overflow=Wrap  en=off  latency=8  dbl_ovrd=off  use_behavioral_HDL=off  opt=Speed  use_embedded=off  optimum_pipeline=on  pipeline=on  use_rpm=on  placement_style=Triangular  block_type=mult
  Register : xbsIndex_r4/Register  init=0  rst=off  en=off  dbl_ovrd=off  block_type=register
  Out1 : Outport
  vld_out : Outport  Port=2
  wires:
  Kx_tbt/1 -> Cast_truncate1/1(In1)
  In1/1 -> Kx_tbt/1
  Cast_truncate1/1(Out1) -> Register/1
  In2/1 -> Kx_tbt/2
  Register/1 -> Out1/1
  vld_in/1 -> Delay1/1
  Delay1/1 -> vld_out/1

== system ddc_bpm_476_066/Ksum_monit_mult2 ==
  In1 : Inport
  In2 : Inport  Port=2
  vld_in : Inport  Port=3
  Cast_truncate1 : Subsystem
  Delay1 : xbsIndex_r4/Delay  rst=off  infoeditControl=Selection of Reset will increase slice count due to use of real FFs and instead of SRLs  en=off  latency=9  dbl_ovrd=off  reg_retiming=off  block_type=delay
  Kx_tbt : xbsIndex_r4/Mult  precision=Full  arith_type="Signed  (2's comp)"  n_bits=16  bin_pt=14  quantization=Truncate  overflow=Wrap  en=off  latency=8  dbl_ovrd=off  use_behavioral_HDL=off  opt=Speed  use_embedded=off  optimum_pipeline=on  pipeline=on  use_rpm=on  placement_style=Triangular  block_type=mult
  Register : xbsIndex_r4/Register  init=0  rst=off  en=off  dbl_ovrd=off  block_type=register
  Out1 : Outport
  vld_out : Outport  Port=2
  wires:
  Kx_tbt/1 -> Cast_truncate1/1(In1)
  In1/1 -> Kx_tbt/1
  Cast_truncate1/1(Out1) -> Register/1
  In2/1 -> Kx_tbt/2
  Register/1 -> Out1/1
  vld_in/1 -> Delay1/1
  Delay1/1 -> vld_out/1

== system ddc_bpm_476_066/Ksum_tbt_mult3 ==
  In1 : Inport
  In2 : Inport  Port=2
  vld_in : Inport  Port=3
  Cast_truncate1 : Subsystem
  Delay1 : xbsIndex_r4/Delay  rst=off  infoeditControl=Selection of Reset will increase slice count due to use of real FFs and instead of SRLs  en=off  latency=9  dbl_ovrd=off  reg_retiming=off  block_type=delay
  Kx_tbt : xbsIndex_r4/Mult  precision=Full  arith_type="Signed  (2's comp)"  n_bits=16  bin_pt=14  quantization=Truncate  overflow=Wrap  en=off  latency=8  dbl_ovrd=off  use_behavioral_HDL=off  opt=Speed  use_embedded=off  optimum_pipeline=on  pipeline=on  use_rpm=on  placement_style=Triangular  block_type=mult
  Register : xbsIndex_r4/Register  init=0  rst=off  en=off  dbl_ovrd=off  block_type=register
  Out1 : Outport
  vld_out : Outport  Port=2
  wires:
  Kx_tbt/1 -> Cast_truncate1/1(In1)
  In1/1 -> Kx_tbt/1
  Cast_truncate1/1(Out1) -> Register/1
  In2/1 -> Kx_tbt/2
  Register/1 -> Out1/1
  vld_in/1 -> Delay1/1
  Delay1/1 -> vld_out/1

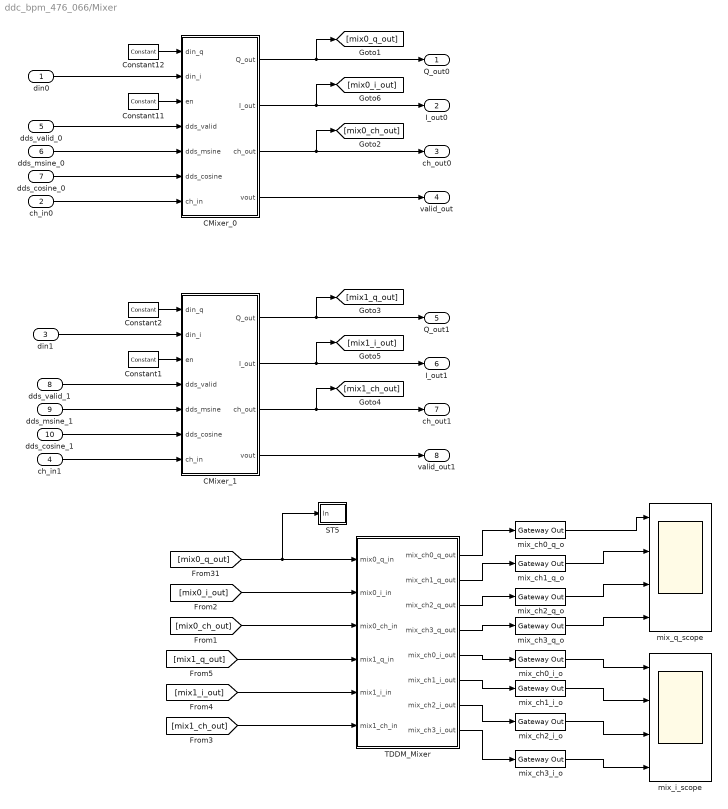
== system ddc_bpm_476_066/Mixer ==
  din0 : Inport
  ch_in0 : Inport  Port=2
  din1 : Inport  Port=3
  ch_in1 : Inport  Port=4
  dds_valid_0 : Inport  Port=5
  dds_msine_0 : Inport  Port=6
  dds_cosine_0 : Inport  Port=7
  dds_valid_1 : Inport  Port=8
  dds_msine_1 : Inport  Port=9
  dds_cosine_1 : Inport  Port=10
  CMixer_0 : Subsystem
  CMixer_1 : Subsystem
  Constant1 : xbsIndex_r4/Constant  const=1  gui_display_data_type=Boolean  arith_type=Boolean  n_bits=24  bin_pt=22  preci_type=Single  exp_width=8  frac_width=24  explicit_period=on  period=dt_sim  equ=P=C  opselect=C  inp2=PCIN>>17  opr=+  inp1=P  carry=CIN  dbl_ovrd=off  block_type=constant
  Constant11 : xbsIndex_r4/Constant  const=1  gui_display_data_type=Boolean  arith_type=Boolean  n_bits=24  bin_pt=22  preci_type=Single  exp_width=8  frac_width=24  explicit_period=on  period=dt_sim  equ=P=C  opselect=C  inp2=PCIN>>17  opr=+  inp1=P  carry=CIN  dbl_ovrd=off  block_type=constant
  Constant12 : xbsIndex_r4/Constant  const=0  gui_display_data_type=Fixed-point  arith_type=Signed (2's comp)  n_bits=24  bin_pt=22  preci_type=Single  exp_width=8  frac_width=24  explicit_period=on  period=dt_sim  equ=P=C  opselect=C  inp2=PCIN>>17  opr=+  inp1=P  carry=CIN  dbl_ovrd=off  block_type=constant
  Constant2 : xbsIndex_r4/Constant  const=0  gui_display_data_type=Fixed-point  arith_type=Signed (2's comp)  n_bits=24  bin_pt=22  preci_type=Single  exp_width=8  frac_width=24  explicit_period=on  period=dt_sim  equ=P=C  opselect=C  inp2=PCIN>>17  opr=+  inp1=P  carry=CIN  dbl_ovrd=off  block_type=constant
  ST5 : Subsystem
  TDDM_Mixer : Subsystem
  mix_ch0_i_o : xbsIndex_r4/Gateway Out  inherit_from_input=on  hdl_port=on  timing_constraint=Data Rate  locs_specified=off  LOCs={}  UseAsDAC=off  DACChannel='1'  block_type=gatewayout
      settings: infoedit="Gateway out block.  Converts Xilinx fixed-point or floating-point type inputs into ouputs of type Simulink integer, single, double, or fixed point.<br><br>Hardware notes:  In hardware these blocks become top level output ports or are discarded, depending on how they are configured."
  mix_ch0_q_o : xbsIndex_r4/Gateway Out  inherit_from_input=on  hdl_port=on  timing_constraint=Data Rate  locs_specified=off  LOCs={}  UseAsDAC=off  DACChannel='1'  block_type=gatewayout
      settings: infoedit="Gateway out block.  Converts Xilinx fixed-point or floating-point type inputs into ouputs of type Simulink integer, single, double, or fixed point.<br><br>Hardware notes:  In hardware these blocks become top level output ports or are discarded, depending on how they are configured."
  mix_ch1_i_o : xbsIndex_r4/Gateway Out  inherit_from_input=on  hdl_port=on  timing_constraint=Data Rate  locs_specified=off  LOCs={}  UseAsDAC=off  DACChannel='1'  block_type=gatewayout
      settings: infoedit="Gateway out block.  Converts Xilinx fixed-point or floating-point type inputs into ouputs of type Simulink integer, single, double, or fixed point.<br><br>Hardware notes:  In hardware these blocks become top level output ports or are discarded, depending on how they are configured."
  mix_ch1_q_o : xbsIndex_r4/Gateway Out  inherit_from_input=on  hdl_port=on  timing_constraint=Data Rate  locs_specified=off  LOCs={}  UseAsDAC=off  DACChannel='1'  block_type=gatewayout
      settings: infoedit="Gateway out block.  Converts Xilinx fixed-point or floating-point type inputs into ouputs of type Simulink integer, single, double, or fixed point.<br><br>Hardware notes:  In hardware these blocks become top level output ports or are discarded, depending on how they are configured."
  mix_ch2_i_o : xbsIndex_r4/Gateway Out  inherit_from_input=on  hdl_port=on  timing_constraint=Data Rate  locs_specified=off  LOCs={}  UseAsDAC=off  DACChannel='1'  block_type=gatewayout
      settings: infoedit="Gateway out block.  Converts Xilinx fixed-point or floating-point type inputs into ouputs of type Simulink integer, single, double, or fixed point.<br><br>Hardware notes:  In hardware these blocks become top level output ports or are discarded, depending on how they are configured."
  mix_ch2_q_o : xbsIndex_r4/Gateway Out  inherit_from_input=on  hdl_port=on  timing_constraint=Data Rate  locs_specified=off  LOCs={}  UseAsDAC=off  DACChannel='1'  block_type=gatewayout
      settings: infoedit="Gateway out block.  Converts Xilinx fixed-point or floating-point type inputs into ouputs of type Simulink integer, single, double, or fixed point.<br><br>Hardware notes:  In hardware these blocks become top level output ports or are discarded, depending on how they are configured."
  mix_ch3_i_o : xbsIndex_r4/Gateway Out  inherit_from_input=on  hdl_port=on  timing_constraint=Data Rate  locs_specified=off  LOCs={}  UseAsDAC=off  DACChannel='1'  block_type=gatewayout
      settings: infoedit="Gateway out block.  Converts Xilinx fixed-point or floating-point type inputs into ouputs of type Simulink integer, single, double, or fixed point.<br><br>Hardware notes:  In hardware these blocks become top level output ports or are discarded, depending on how they are configured."
  mix_ch3_q_o : xbsIndex_r4/Gateway Out  inherit_from_input=on  hdl_port=on  timing_constraint=Data Rate  locs_specified=off  LOCs={}  UseAsDAC=off  DACChannel='1'  block_type=gatewayout
      settings: infoedit="Gateway out block.  Converts Xilinx fixed-point or floating-point type inputs into ouputs of type Simulink integer, single, double, or fixed point.<br><br>Hardware notes:  In hardware these blocks become top level output ports or are discarded, depending on how they are configured."
  mix_i_scope : Scope  NumInputPorts=4
      settings: TimeRange=0.00011214  YMin=-0.1~-1.5~-0.002~-1.5  YMax=1~1.5~0.00075~1.5  SaveName=ScopeData14  MaxDataPoints=1000000  SampleInput=on
  mix_q_scope : Scope  NumInputPorts=4
      settings: TimeRange=0.00011214  YMin=-0.1~-1.5~-0.002~-1.5  YMax=1~1.5~0.00075~1.5  SaveName=ScopeData13  MaxDataPoints=1000000  SampleInput=on
  Q_out0 : Outport
  I_out0 : Outport  Port=2
  ch_out0 : Outport  Port=3
  valid_out : Outport  Port=4
  Q_out1 : Outport  Port=5
  I_out1 : Outport  Port=6
  ch_out1 : Outport  Port=7
  valid_out1 : Outport  Port=8
  wires:
  Constant12/1 -> CMixer_0/1(din_q)
  Constant11/1 -> CMixer_0/3(en)
  CMixer_0/1(Q_out) -> Q_out0/1, [mix0_q_out]
  din0/1 -> CMixer_0/2(din_i)
  CMixer_0/2(I_out) -> I_out0/1, [mix0_i_out]
  dds_valid_0/1 -> CMixer_0/4(dds_valid)
  dds_cosine_0/1 -> CMixer_0/6(dds_cosine)
  CMixer_0/3(ch_out) -> ch_out0/1, [mix0_ch_out]
  dds_msine_0/1 -> CMixer_0/5(dds_msine)
  CMixer_0/4(vout) -> valid_out/1
  ch_in0/1 -> CMixer_0/7(ch_in)
  [mix0_q_out] -> TDDM_Mixer/1(mix0_q_in), ST5/1(In)
  [mix0_ch_out] -> TDDM_Mixer/3(mix0_ch_in)
  [mix0_i_out] -> TDDM_Mixer/2(mix0_i_in)
  TDDM_Mixer/1(mix_ch0_q_out) -> mix_ch0_q_o/1
  TDDM_Mixer/2(mix_ch1_q_out) -> mix_ch1_q_o/1
  TDDM_Mixer/3(mix_ch2_q_out) -> mix_ch2_q_o/1
  TDDM_Mixer/4(mix_ch3_q_out) -> mix_ch3_q_o/1
  TDDM_Mixer/5(mix_ch0_i_out) -> mix_ch0_i_o/1
  TDDM_Mixer/6(mix_ch1_i_out) -> mix_ch1_i_o/1
  TDDM_Mixer/7(mix_ch2_i_out) -> mix_ch2_i_o/1
  TDDM_Mixer/8(mix_ch3_i_out) -> mix_ch3_i_o/1
  mix_ch0_i_o/1 -> mix_i_scope/1
  mix_ch1_i_o/1 -> mix_i_scope/2
  mix_ch2_i_o/1 -> mix_i_scope/3
  mix_ch3_i_o/1 -> mix_i_scope/4
  mix_ch3_q_o/1 -> mix_q_scope/4
  mix_ch2_q_o/1 -> mix_q_scope/3
  mix_ch1_q_o/1 -> mix_q_scope/2
  mix_ch0_q_o/1 -> mix_q_scope/1
  Constant2/1 -> CMixer_1/1(din_q)
  Constant1/1 -> CMixer_1/3(en)
  CMixer_1/1(Q_out) -> Q_out1/1, [mix1_q_out]
  din1/1 -> CMixer_1/2(din_i)
  CMixer_1/2(I_out) -> I_out1/1, [mix1_i_out]
  CMixer_1/3(ch_out) -> ch_out1/1, [mix1_ch_out]
  CMixer_1/4(vout) -> valid_out1/1
  ch_in1/1 -> CMixer_1/7(ch_in)
  [mix1_q_out] -> TDDM_Mixer/4(mix1_q_in)
  [mix1_i_out] -> TDDM_Mixer/5(mix1_i_in)
  [mix1_ch_out] -> TDDM_Mixer/6(mix1_ch_in)
  dds_valid_1/1 -> CMixer_1/4(dds_valid)
  dds_msine_1/1 -> CMixer_1/5(dds_msine)
  dds_cosine_1/1 -> CMixer_1/6(dds_cosine)

== system ddc_bpm_476_066/Monit_amp ==
  din : Inport
  ch_in : Inport  Port=2
  Monit_amp_c : Subsystem
  TDDM_monit_amp_out : Subsystem
  Terminator5 : Terminator
  amp_out0 : Outport
  amp_out1 : Outport  Port=2
  amp_out2 : Outport  Port=3
  amp_out3 : Outport  Port=4
  wires:
  Monit_amp_c/1(amp_out) -> TDDM_monit_amp_out/1(monit_amp_din)
  Monit_amp_c/2(ch_out) -> TDDM_monit_amp_out/2(monit_amp_ch_in)
  Monit_amp_c/3(valid_out) -> Terminator5/1
  TDDM_monit_amp_out/1(monit_amp_data0_out) -> amp_out0/1
  din/1 -> Monit_amp_c/1(din)
  TDDM_monit_amp_out/2(monit_amp_data1_out) -> amp_out1/1
  TDDM_monit_amp_out/3(monit_amp_data2_out) -> amp_out2/1
  ch_in/1 -> Monit_amp_c/2(ch_in)
  TDDM_monit_amp_out/4(monit_amp_data3_out) -> amp_out3/1

== system ddc_bpm_476_066/ST1 ==
  In : Inport
  Display : Display
  Sample Time : xbsIndex_r4/Sample Time  block_type=sampletime
      settings: infoedit="The Sample Time block reports the normalized sample period of its input.  A signal's normalized sample period is not equivalent to its Simulink absolute sample period.<br><br>Hardware notes: This block is implemented as a constant in hardware."
  out : xbsIndex_r4/Gateway Out  inherit_from_input=on  hdl_port=off  timing_constraint=Data Rate  locs_specified=off  LOCs={}  UseAsDAC=off  DACChannel='1'  block_type=gatewayout
      settings: infoedit="Gateway out block.  Converts Xilinx fixed-point or floating-point type inputs into ouputs of type Simulink integer, single, double, or fixed point.<br><br>Hardware notes:  In hardware these blocks become top level output ports or are discarded, depending on how they are configured."
  wires:
  out/1 -> Display/1
  Sample Time/1 -> out/1
  In/1 -> Sample Time/1

== system ddc_bpm_476_066/ST10 ==
  In : Inport
  Display : Display
  Sample Time : xbsIndex_r4/Sample Time  block_type=sampletime
      settings: infoedit="The Sample Time block reports the normalized sample period of its input.  A signal's normalized sample period is not equivalent to its Simulink absolute sample period.<br><br>Hardware notes: This block is implemented as a constant in hardware."
  out : xbsIndex_r4/Gateway Out  inherit_from_input=on  hdl_port=off  timing_constraint=Data Rate  locs_specified=off  LOCs={}  UseAsDAC=off  DACChannel='1'  block_type=gatewayout
      settings: infoedit="Gateway out block.  Converts Xilinx fixed-point or floating-point type inputs into ouputs of type Simulink integer, single, double, or fixed point.<br><br>Hardware notes:  In hardware these blocks become top level output ports or are discarded, depending on how they are configured."
  wires:
  out/1 -> Display/1
  Sample Time/1 -> out/1
  In/1 -> Sample Time/1

== system ddc_bpm_476_066/ST2 ==
  In : Inport
  Display : Display
  Sample Time : xbsIndex_r4/Sample Time  block_type=sampletime
      settings: infoedit="The Sample Time block reports the normalized sample period of its input.  A signal's normalized sample period is not equivalent to its Simulink absolute sample period.<br><br>Hardware notes: This block is implemented as a constant in hardware."
  out : xbsIndex_r4/Gateway Out  inherit_from_input=on  hdl_port=off  timing_constraint=Data Rate  locs_specified=off  LOCs={}  UseAsDAC=off  DACChannel='1'  block_type=gatewayout
      settings: infoedit="Gateway out block.  Converts Xilinx fixed-point or floating-point type inputs into ouputs of type Simulink integer, single, double, or fixed point.<br><br>Hardware notes:  In hardware these blocks become top level output ports or are discarded, depending on how they are configured."
  wires:
  out/1 -> Display/1
  Sample Time/1 -> out/1
  In/1 -> Sample Time/1
